simulink model "Planta"  (R2019a)
settings: Solver=VariableStepAuto  StartTime=0.0  StopTime=60  RelTol=1e-3
settings Model: Creator=Alejoxbg  LastModifiedBy=Alejoxbg

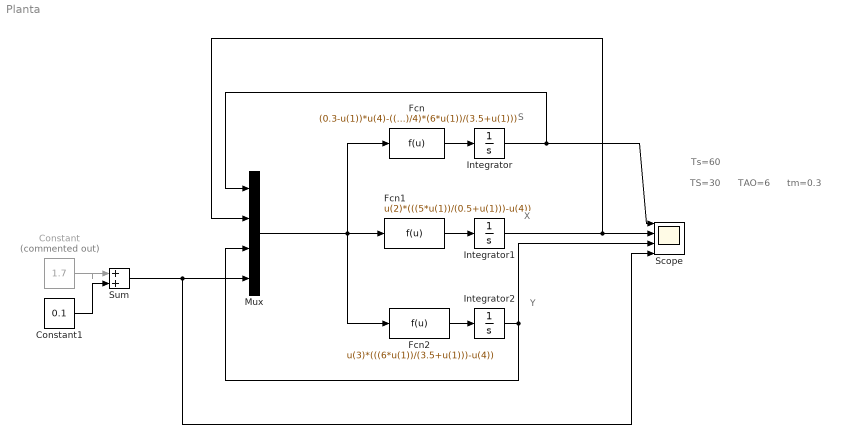
== system Planta ==
  note: TAO=6
  note: tm=0.3
  note: TS=30
  note: Ts=60
  note: Y
  note: X
  note: S
  Constant : Constant  Commented=on  Value=1.7
  Constant1 : Constant  Value=0.1
  Fcn : Fcn  Expr=(0.3-u(1))*u(4)-((u(2)/4)*(5*u(1))/(0.5+u(1)))-((u(3)/4)*(6*u(1))/(3.5+u(1)))
  Fcn1 : Fcn  Expr=u(2)*(((5*u(1))/(0.5+u(1)))-u(4))
  Fcn2 : Fcn  Expr=u(3)*(((6*u(1))/(3.5+u(1)))-u(4))
  Integrator : Integrator
  Integrator1 : Integrator  InitialCondition=0.1
  Integrator2 : Integrator
  Mux : Mux
  Scope : Scope  NumInputPorts=4
  Sum : Sum  Inputs=|++
  wires:
  Mux/1 -> Fcn/1, Fcn1/1, Fcn2/1
  Fcn/1 -> Integrator/1
  Fcn1/1 -> Integrator1/1
  Fcn2/1 -> Integrator2/1
  Integrator/1 -> Scope/1, Mux/1
  Integrator1/1 -> Mux/2, Scope/2
  Integrator2/1 -> Mux/3, Scope/3
  Sum/1 -> Scope/4, Mux/4
  Constant/1 -> Sum/1
  Constant1/1 -> Sum/2
